simulink model "counter_9"  (R2018a)
settings: Solver=FixedStepAuto  StartTime=0.0  StopTime=10.0  RelTol=1e-3
settings Model: Creator=SONY  LastModifiedBy=SONY

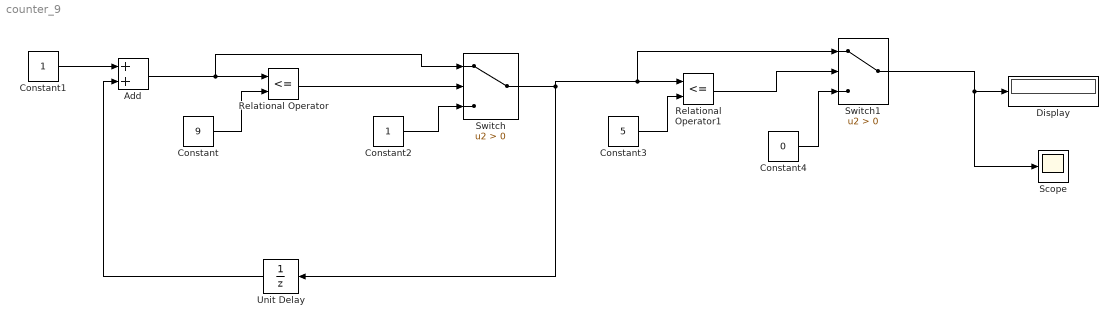
== system counter_9 ==
  Add : Sum
  Constant : Constant  Value=9
  Constant1 : Constant
  Constant2 : Constant
  Constant3 : Constant  Value=5
  Constant4 : Constant  Value=0
  Display : Display
  Relational Operator : RelationalOperator  Operator=<=  OutDataTypeStr=boolean  RndMeth=Simplest
  Relational Operator1 : RelationalOperator  Operator=<=  OutDataTypeStr=boolean  RndMeth=Simplest
  Scope : Scope
  Switch : Switch  Criteria=u2 > Threshold
  Switch1 : Switch  Criteria=u2 > Threshold
  Unit Delay : UnitDelay  InitialCondition=-1  SampleTime=-1
  wires:
  Constant1/1 -> Add/1
  Constant/1 -> Relational Operator/2
  Add/1 -> Switch/1, Relational Operator/1
  Constant2/1 -> Switch/3
  Relational Operator/1 -> Switch/2
  Switch/1 -> Switch1/1, Relational Operator1/1, Unit Delay/1
  Unit Delay/1 -> Add/2
  Relational Operator1/1 -> Switch1/2
  Switch1/1 -> Scope/1, Display/1
  Constant3/1 -> Relational Operator1/2
  Constant4/1 -> Switch1/3
